simulink subsystem "Pose_Publisher"  (R2022b)
settings: Solver=VariableStepAuto  StartTime=0.0  StopTime=10.0  RelTol=1e-3
undefined symbols (not defined in the file or in its folder): header, pose
libraries: ros2lib x2
settings Model: Creator=hayden  LastModifiedBy=hollis
settings ModelReferenceCC: EnableRefExpFcnMdlSchedulingChecks=on

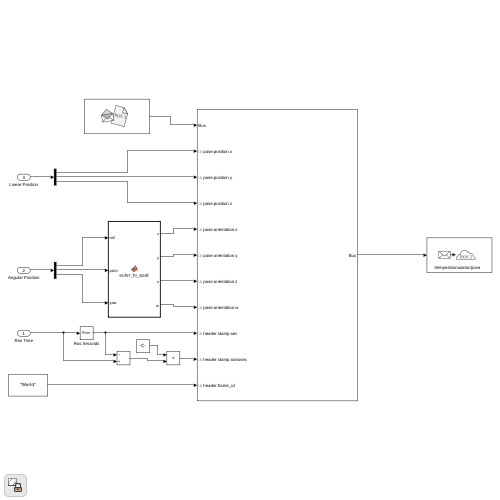
[thumbnail: Simulink's stored preview of the top-level diagram]
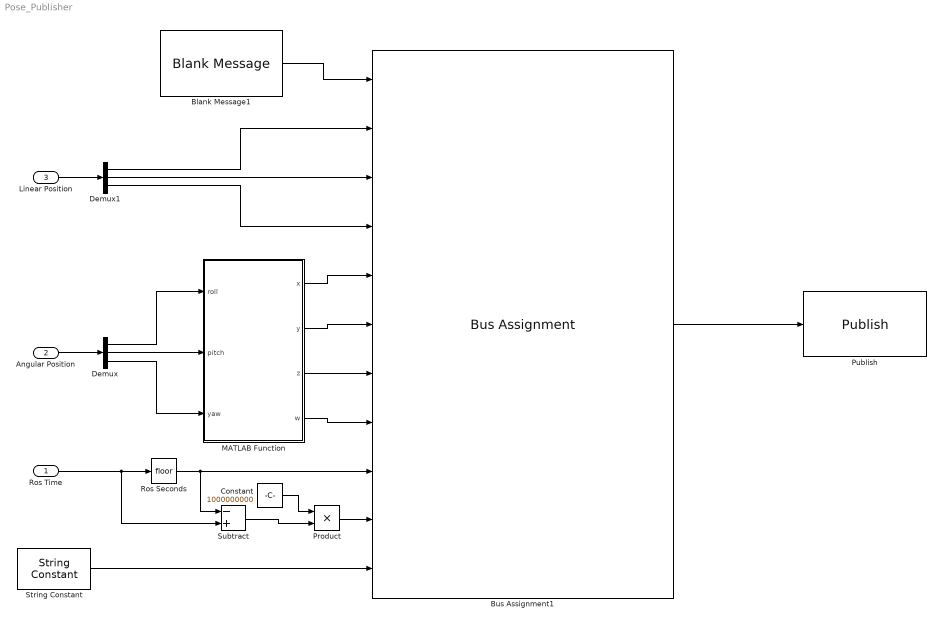
== system Pose_Publisher ==
  Ros Time : Inport
  Angular Position : Inport  Port=2
  Linear Position : Inport  Port=3
  Blank Message1 : ros2lib/Blank Message  messageClass=Message  entityType=geometry_msgs/PoseStamped  messageType=geometry_msgs/PoseStamped  SampleTime=inf
  Bus Assignment1 : BusAssignment  AssignedSignals=pose.position.x,pose.position.y,pose.position.z,pose.orientation.x,pose.orientation.y,pose.orientation.z,pose.orientation.w,header.stamp.sec,header.stamp.nanosec,header.frame_id
  Constant : Constant  Value=1000000000
  Demux : Demux  Outputs=3
  Demux1 : Demux  Outputs=3
  MATLAB Function : MATLAB Function  TreatAsAtomicUnit=on
  Product : Product
  Publish : ros2lib/Publish  topicSource=Select from ROS network  topic=/tempest/simulator/pose  messageType=geometry_msgs/Pose  QOSHistory=Keep last  QOSDepth=1  QOSReliability=Reliable  QOSDurability=Volatile
  Ros Seconds : Rounding
  String Constant : StringConstant  String="\"World\""
  Subtract : Sum  Inputs=-+
  wires:
  Blank Message1/1 -> Bus Assignment1/1
  MATLAB Function/1(x) -> Bus Assignment1/5
  MATLAB Function/2(y) -> Bus Assignment1/6
  MATLAB Function/3(z) -> Bus Assignment1/7
  MATLAB Function/4(w) -> Bus Assignment1/8
  Bus Assignment1/1 -> Publish/1
  Demux/2 -> MATLAB Function/2(pitch)
  Demux/1 -> MATLAB Function/1(roll)
  Demux/3 -> MATLAB Function/3(yaw)
  Angular Position/1 -> Demux/1
  Linear Position/1 -> Demux1/1
  Demux1/1 -> Bus Assignment1/2
  Demux1/2 -> Bus Assignment1/3
  Demux1/3 -> Bus Assignment1/4
  Ros Time/1 -> Ros Seconds/1, Subtract/2
  Ros Seconds/1 -> Bus Assignment1/9, Subtract/1
  Product/1 -> Bus Assignment1/10
  Subtract/1 -> Product/2
  Constant/1 -> Product/1
  String Constant/1 -> Bus Assignment1/11

== matlab function Pose_Publisher/MATLAB Function ==
  data: roll input; x output; pitch input; yaw input; y output; z output; w output
function [x,y,z,w]= euler_to_quat(roll, pitch, yaw)
    euler = [roll, pitch, yaw];
    SEQ = "XYZ";
    quat = eul2quat(euler, SEQ);
    x = quat(1);
    y = quat(2);
    z = quat(3);
    w = quat(4);
